simulink model "model_v2"  (R2016b)
settings: Solver=ode45  StartTime=0.0  StopTime=10  RelTol=1e-3  EnableMultiTasking=on
model workspace: external: MATLAB File par_struct.m (data not in the file)
values from neighbouring files (symbols this model uses):
  par = struct    [par_struct.m]
  torque_bypass = 0    [parameters.m]
undefined symbols (not defined in the file or in its folder): initial_state
settings Model: Creator=Nathan  LastModifiedBy=Ortix
settings DataIOCC: InitialState=states  LimitDataPoints=on  SaveFormat=Array
settings OptimizationCC: LifeSpan=inf
settings DebuggingCC: AllowSymbolicDim=off  SFUnexpectedBacktrackingDiag=warning  SFNoUnconditionalDefaultTransitionDiag=warning  SFExecutionAtInitializationDiag=none
settings HardwareCC: ProdBitPerPointer=32  ProdBitPerSizeT=32  ProdBitPerPtrDiffT=32  ProdLargestAtomicFloat=None  ProdIntDivRoundTo=Undefined  ProdEndianess=Unspecified  ProdWordSize=32  ProdHWDeviceType=32-bit Generic
settings ModelReferenceCC: PropagateSignalLabelsOutOfModel=off
settings GRTTargetCC: TargetLangStandard=C89/C90 (ANSI)  GeneratePreprocessorConditionals=Disable all
settings ConfigComp: CovMetricSettings=dw  CovHtmlReporting=on  CovSaveCumulativeToWorkspaceVar=on  CovSaveSingleToWorkspaceVar=on  CovExternalEMLEnable=off

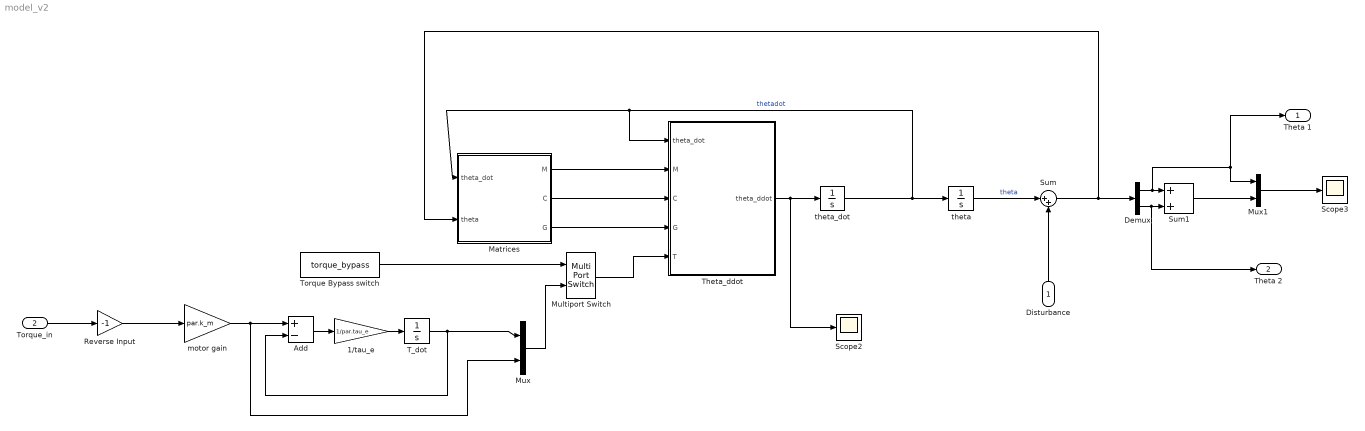
== system model_v2 ==
  Disturbance : Inport  PortDimensions=2
  Torque_in : Inport  Port=2
  "1/tau_e " : Gain  Gain=1/par.tau_e
  Add : Sum  Inputs=+-
  Demux : Demux  Outputs=2
  Matrices : MATLAB Function  TreatAsAtomicUnit=on
  Multiport Switch : MultiPortSwitch  DataPortOrder=Zero-based contiguous  Inputs=1
  Mux : Mux  Inputs=2
  Mux1 : Mux  Inputs=2
  Reverse Input : Gain  Gain=-1
  Scope2 : Scope
  Scope3 : Scope
  Sum : Sum  Inputs=|++
  Sum1 : Sum
  T_dot : Integrator
  "Theta_ddot " : MATLAB Function  TreatAsAtomicUnit=on
  Torque Bypass switch : Constant  Value=torque_bypass
  "motor gain " : Gain  Gain=par.k_m
  "theta " : Integrator  InitialCondition=initial_state
  "theta_dot " : Integrator
  Theta 1 : Outport
  Theta 2 : Outport  Port=2
  wires:
  Torque_in/1 -> Reverse Input/1
  T_dot/1 -> Add/2, Mux/1
  "theta_dot "/1 -> "theta "/1, "Theta_ddot "/1(theta_dot), Matrices/1(theta_dot)  "thetadot"
  Matrices/3(G) -> "Theta_ddot "/4(G)
  Matrices/1(M) -> "Theta_ddot "/2(M)
  "Theta_ddot "/1(theta_ddot) -> Scope2/1, "theta_dot "/1
  Matrices/2(C) -> "Theta_ddot "/3(C)
  Add/1 -> "1/tau_e "/1
  "1/tau_e "/1 -> T_dot/1
  "theta "/1 -> Sum/1  "theta"
  Mux/1 -> Multiport Switch/2
  Torque Bypass switch/1 -> Multiport Switch/1
  "motor gain "/1 -> Mux/2, Add/1
  Demux/1 -> Theta 1/1, Mux1/1, Sum1/1
  Demux/2 -> Theta 2/1, Sum1/2
  Reverse Input/1 -> "motor gain "/1
  Sum1/1 -> Mux1/2
  Sum/1 -> Matrices/2(theta), Demux/1
  Mux1/1 -> Scope3/1
  Multiport Switch/1 -> "Theta_ddot "/5(T)
  Disturbance/1 -> Sum/2

== matlab function model_v2/Theta_ddot  ==
  data: theta_dot input; M input; C input; G input; theta_ddot output; T input
function theta_ddot = fcn(theta_dot,M,C,G,T)
theta_ddot = [0;0];

theta_ddot = M\[T;0] - M\C*theta_dot - M\G;

== matlab function model_v2/Matrices ==
  data: theta_dot input; theta input; M output; C output; G output
function [M, C, G] = fcn(theta_dot, theta)

M = zeros(2);
C = zeros(2);
G = [0;0];

g = 9.81; 
l1 = 0.1;
l2 = 0.1;
m1 = 0.125;
m2 = 0.05;
c1 = -0.04;
c2 = 0.06;
I1 = 0.074;
I2 = 0.00012;
b1 = 4.8;
b2 = 0.0002;

P1 = m1*c1^2+m2*l1^2+I1;
P2 = m2*c2^2+ I2;
P3 = m2*l1*c2;
g1 = (m1*c1+m2*l1)*g;
g2 = m2*c2*g;

M = [(P1 + P2 + 2*P3*cos(theta(2)))               (P2 + P3*cos(theta(2))) ;
     (P2 + P3*cos(theta(2)))                       P2                   ];
 
 
C = [(b1 - P3*theta_dot(2)*sin(theta(2)))           (-P3*(theta_dot(1)+theta_dot(2))*sin(theta(2))) ;
     (P3*theta_dot(1)*sin(theta(2)))                 b2                                      ];
     
G = [(-g1*sin(theta(1))-g2*sin(theta(1) + theta(2))) ;
      -g2*sin(theta(1)+theta(2))                   ];
% function [M, C, G] = fcn(theta_dot, theta, par)
% 
% M = zeros(2);
% C = zeros(2);
% G = [0;0];
% 
% 
% M = [(par.P1 + par.P2 + 2*par.P3*cos(theta(2))) (par.P2 + par.P3*cos(theta(2))) ;
%     (par.P2 + par.P3*cos(theta(2)))                       par.P2               ];
% 
% 
% C = [(par.b1 - par.P3*theta_dot(2)*sin(theta(2))) (-par.P3*(theta_dot(1)+theta_dot(2))*sin(theta(2))) ;
%     (par.P3*theta_dot(1)*sin(theta(2)))                 par.b2          ];
% 
% G = [(-par.g1*sin(theta(1))-par.g2*sin(theta(1) + theta(2))) ;
%     -par.g2*sin(theta(1)+theta(2))                   ];
